simulink model "model_all"  (R2020a)
settings: Solver=VariableStepAuto  StartTime=0.0  StopTime=10.0  RelTol=1e-3
values from neighbouring files (symbols this model uses):
  delta_max = 20    [initialize_all.m]
  ir = 1.7    [initialize_all.m]
  parking_speed = 0.1    [initialize_all.m]
  pr = 1.3    [initialize_all.m]
  TOF_distance_limit = 20    [initialize_all.m]
undefined symbols (not defined in the file or in its folder): denom_drehzahl, num_drehzahl
libraries: robotlib x20, simulink x4, drivingvehiclecontroller x2

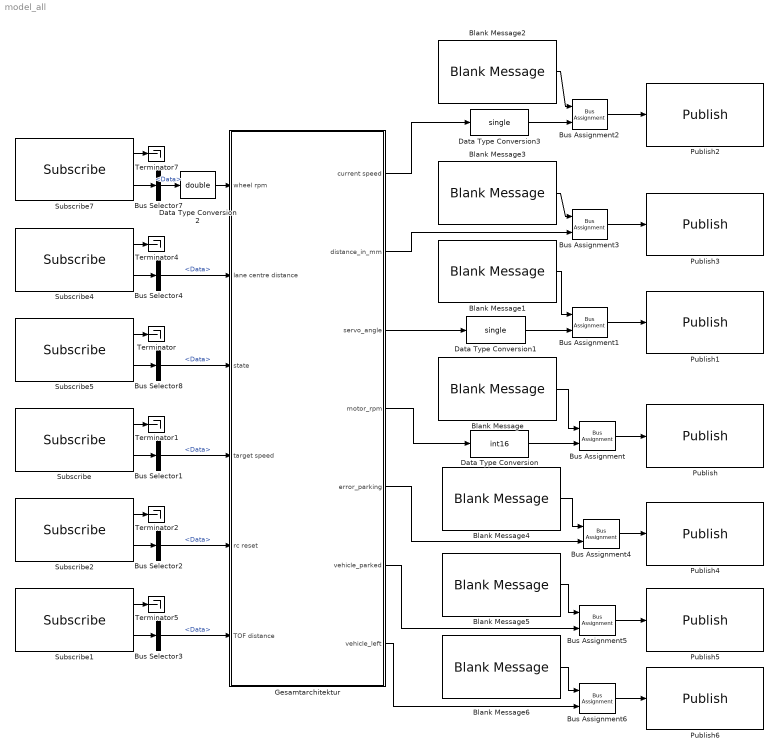
== system model_all ==
  Blank Message : robotlib/Blank Message  messageClass=Message  entityType=std_msgs/Int16  messageType=std_msgs/Int16  SampleTime=inf
  Blank Message1 : robotlib/Blank Message  messageClass=Message  entityType=std_msgs/Float32  messageType=std_msgs/Float32  SampleTime=inf
  Blank Message2 : robotlib/Blank Message  messageClass=Message  entityType=std_msgs/Float32  messageType=std_msgs/Float32  SampleTime=inf
  Blank Message3 : robotlib/Blank Message  messageClass=Message  entityType=std_msgs/Float32  messageType=std_msgs/Float32  SampleTime=inf
  Blank Message4 : robotlib/Blank Message  messageClass=Message  entityType=std_msgs/Bool  messageType=std_msgs/Bool  SampleTime=inf
  Blank Message5 : robotlib/Blank Message  messageClass=Message  entityType=std_msgs/Bool  messageType=std_msgs/Bool  SampleTime=inf
  Blank Message6 : robotlib/Blank Message  messageClass=Message  entityType=std_msgs/Bool  messageType=std_msgs/Bool  SampleTime=inf
  Bus Assignment{,1..6} (7 alike) : BusAssignment  AssignedSignals=Data
  Bus Selector{1..4,7..8} (6 alike) : BusSelector  OutputSignals=Data
  Data Type Conversion : DataTypeConversion  OutDataTypeStr=int16
  Data Type Conversion1 : DataTypeConversion  OutDataTypeStr=single
  Data Type Conversion2 : DataTypeConversion  OutDataTypeStr=double
  Data Type Conversion3 : DataTypeConversion  OutDataTypeStr=single
  Gesamtarchitektur : Subsystem
  Publish : robotlib/Publish  topicSource=Specify your own  topic=/ctl_motorRpm  messageType=std_msgs/Int16  messageQueueLength=1
  Publish1 : robotlib/Publish  topicSource=Specify your own  topic=/ctl_servoAngle  messageType=std_msgs/Float32  messageQueueLength=1
  Publish2 : robotlib/Publish  topicSource=Specify your own  topic=/ctl_velocity  messageType=std_msgs/Float32  messageQueueLength=1
  Publish3 : robotlib/Publish  topicSource=Specify your own  topic=/ctl_distance  messageType=std_msgs/Float32  messageQueueLength=1
  Publish4 : robotlib/Publish  topicSource=Specify your own  topic=/ctl_errorParking  messageType=std_msgs/Bool  messageQueueLength=1
  Publish5 : robotlib/Publish  topicSource=Specify your own  topic=/ctl_parked  messageType=std_msgs/Bool  messageQueueLength=1
  Publish6 : robotlib/Publish  topicSource=Specify your own  topic=/ctl_leavedParkingLot  messageType=std_msgs/Bool  messageQueueLength=1
  Subscribe : robotlib/Subscribe  topicSource=Specify your own  topic=/trj_targetSpeed  messageType=std_msgs/Float32  sampleTime=-1  messageQueueLength=1
  Subscribe1 : robotlib/Subscribe  topicSource=Specify your own  topic=/sns_tof_front  messageType=std_msgs/Float32  sampleTime=-1  messageQueueLength=1
  Subscribe2 : robotlib/Subscribe  topicSource=Specify your own  topic=/akt_rc  messageType=std_msgs/Bool  sampleTime=-1  messageQueueLength=1
  Subscribe4 : robotlib/Subscribe  topicSource=Specify your own  topic=/trj_deltaY  messageType=std_msgs/Float32  sampleTime=-1  messageQueueLength=1
  Subscribe5 : robotlib/Subscribe  topicSource=Specify your own  topic=/state  messageType=std_msgs/Int16  sampleTime=-1  messageQueueLength=1
  Subscribe7 : robotlib/Subscribe  topicSource=Specify your own  topic=/sns_wheelRpm  messageType=std_msgs/Float32  sampleTime=-1  messageQueueLength=1
  Terminator{,1..2,4..5,7} (6 alike) : Terminator
  wires:
  Data Type Conversion/1 -> Bus Assignment/2
  Blank Message/1 -> Bus Assignment/1
  Subscribe/1 -> Terminator1/1
  Bus Assignment/1 -> Publish/1
  Subscribe/2 -> Bus Selector1/1
  Subscribe2/2 -> Bus Selector2/1
  Subscribe2/1 -> Terminator2/1
  Bus Assignment1/1 -> Publish1/1
  Blank Message1/1 -> Bus Assignment1/1
  Data Type Conversion1/1 -> Bus Assignment1/2
  Subscribe4/1 -> Terminator4/1
  Subscribe4/2 -> Bus Selector4/1
  Bus Assignment3/1 -> Publish3/1
  Data Type Conversion3/1 -> Bus Assignment2/2
  Bus Assignment2/1 -> Publish2/1
  Subscribe7/1 -> Terminator7/1
  Blank Message3/1 -> Bus Assignment3/1
  Subscribe7/2 -> Bus Selector7/1
  Blank Message2/1 -> Bus Assignment2/1
  Bus Selector7/1 -> Data Type Conversion2/1  "<Data>"
  Subscribe1/2 -> Bus Selector3/1
  Subscribe1/1 -> Terminator5/1
  Subscribe5/1 -> Terminator/1
  Subscribe5/2 -> Bus Selector8/1
  Bus Assignment4/1 -> Publish4/1
  Blank Message4/1 -> Bus Assignment4/1
  Gesamtarchitektur/5(error_parking) -> Bus Assignment4/2
  Blank Message5/1 -> Bus Assignment5/1
  Bus Assignment5/1 -> Publish5/1
  Gesamtarchitektur/6(vehicle_parked) -> Bus Assignment5/2
  Blank Message6/1 -> Bus Assignment6/1
  Bus Assignment6/1 -> Publish6/1
  Gesamtarchitektur/7(vehicle_left) -> Bus Assignment6/2
  Data Type Conversion2/1 -> Gesamtarchitektur/1(wheel rpm)
  Bus Selector4/1 -> Gesamtarchitektur/2(lane centre distance)  "<Data>"
  Bus Selector8/1 -> Gesamtarchitektur/3(state)  "<Data>"
  Bus Selector1/1 -> Gesamtarchitektur/4(target speed)  "<Data>"
  Bus Selector2/1 -> Gesamtarchitektur/5(rc reset)  "<Data>"
  Bus Selector3/1 -> Gesamtarchitektur/6(TOF distance)  "<Data>"
  Gesamtarchitektur/1(current speed) -> Data Type Conversion3/1
  Gesamtarchitektur/2(distance_in_mm) -> Bus Assignment3/2
  Gesamtarchitektur/3(servo_angle) -> Data Type Conversion1/1
  Gesamtarchitektur/4(motor_rpm) -> Data Type Conversion/1

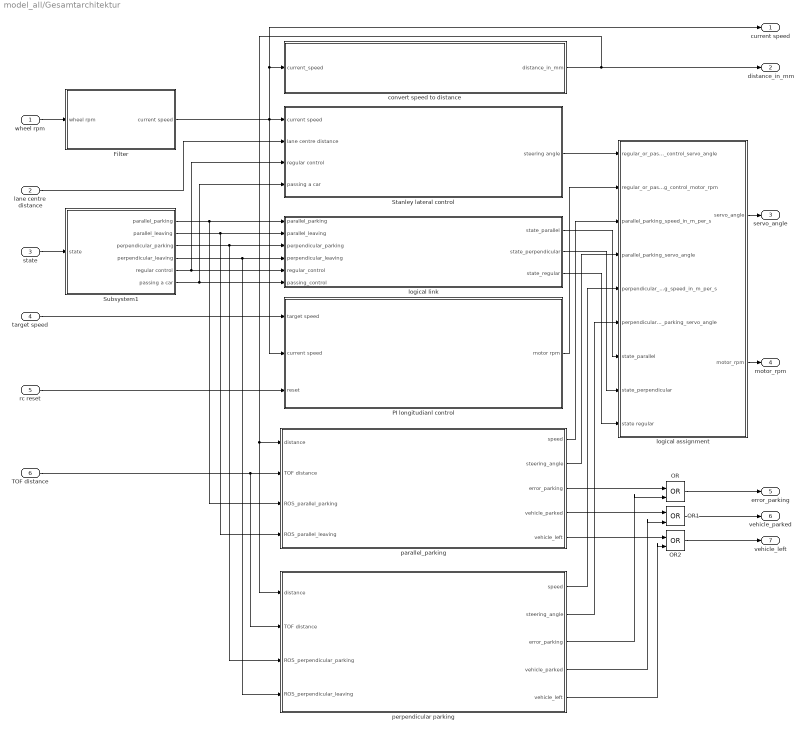
== system model_all/Gesamtarchitektur ==
  wheel rpm : Inport
  lane centre distance : Inport  Port=2
  state : Inport  Port=3
  target speed : Inport  Port=4
  rc reset : Inport  Port=5
  TOF distance : Inport  Port=6
  "Filter " : Subsystem
  OR : Logic  Operator=OR  IconShape=distinctive  AllPortsSameDT=off  OutDataTypeStr=boolean
  OR1 : Logic  Operator=OR  IconShape=distinctive  AllPortsSameDT=off  OutDataTypeStr=boolean
  OR2 : Logic  Operator=OR  IconShape=distinctive  AllPortsSameDT=off  OutDataTypeStr=boolean
  "PI longitudianl control " : Subsystem
  Stanley lateral control : Subsystem
  Subsystem1 : Subsystem
  convert speed to distance : Subsystem
  logical assignment : Subsystem
  logical link : Subsystem
  parallel_parking : Subsystem
  perpendicular parking : Subsystem
  current speed : Outport
  distance_in_mm : Outport  Port=2
  servo_angle : Outport  Port=3
  motor_rpm : Outport  Port=4
  error_parking : Outport  Port=5
  vehicle_parked : Outport  Port=6
  vehicle_left : Outport  Port=7
  wires:
  parallel_parking/1(speed) -> logical assignment/3(parallel_parking_speed_in_m_per_s)
  convert speed to distance/1(distance_in_mm) -> distance_in_mm/1, perpendicular parking/1(distance), parallel_parking/1(distance)
  logical assignment/2(motor_rpm) -> motor_rpm/1
  wheel rpm/1 -> "Filter "/1(wheel rpm)
  TOF distance/1 -> perpendicular parking/2(TOF distance), parallel_parking/2(TOF distance)
  perpendicular parking/1(speed) -> logical assignment/5(perpendicular_parking_speed_in_m_per_s)
  rc reset/1 -> "PI longitudianl control "/3("reset ")
  "Filter "/1(current speed) -> current speed/1, convert speed to distance/1(current_speed), "PI longitudianl control "/2("current speed "), Stanley lateral control/1(current speed)
  Subsystem1/6(passing a car) -> logical link/6(passing_control), Stanley lateral control/4(passing a car)
  state/1 -> Subsystem1/1(state)
  Subsystem1/3(perpendicular_parking) -> perpendicular parking/3(ROS_perpendicular_parking), logical link/3(perpendicular_parking)
  Subsystem1/2(parallel_leaving) -> parallel_parking/4(ROS_parallel_leaving), logical link/2(parallel_leaving)
  Subsystem1/4(perpendicular_leaving) -> logical link/4(perpendicular_leaving), perpendicular parking/4(ROS_perpendicular_leaving)
  Subsystem1/1(parallel_parking) -> parallel_parking/3(ROS_parallel_parking), logical link/1(parallel_parking)
  logical link/2(state_perpendicular) -> logical assignment/8(state_perpendicular)
  Subsystem1/5(regular control) -> Stanley lateral control/3(regular control), logical link/5(regular_control)
  logical link/3(state_regular) -> logical assignment/9(state regular)
  logical link/1(state_parallel) -> logical assignment/7(state_parallel)
  "PI longitudianl control "/1("motor rpm ") -> logical assignment/2(regular_or_passing_control_motor_rpm)
  Stanley lateral control/1(steering angle) -> logical assignment/1(regular_or_passing_control_servo_angle)
  perpendicular parking/2(steering_angle) -> logical assignment/6(perpendicular_parking_servo_angle)
  parallel_parking/2(steering_angle) -> logical assignment/4(parallel_parking_servo_angle)
  logical assignment/1(servo_angle) -> servo_angle/1
  target speed/1 -> "PI longitudianl control "/1("target speed ")
  lane centre distance/1 -> Stanley lateral control/2(lane centre distance)
  perpendicular parking/3(error_parking) -> OR/2
  OR/1 -> error_parking/1
  parallel_parking/3(error_parking) -> OR/1
  OR2/1 -> vehicle_left/1
  perpendicular parking/5(vehicle_left) -> OR2/2
  parallel_parking/5(vehicle_left) -> OR2/1
  perpendicular parking/4(vehicle_parked) -> OR1/2
  OR1/1 -> vehicle_parked/1
  parallel_parking/4(vehicle_parked) -> OR1/1

== system model_all/Gesamtarchitektur/Filter  ==
  wheel rpm : Inport
  Discrete Transfer Fcn : DiscreteTransferFcn  Numerator=num_drehzahl  Denominator=denom_drehzahl
  rpm to 1/s : Gain  Gain=1/60
  wheel radius : Gain  Gain=0.175896
  current speed : Outport
  wires:
  Discrete Transfer Fcn/1 -> wheel radius/1
  wheel rpm/1 -> rpm to 1/s/1
  wheel radius/1 -> current speed/1
  rpm to 1/s/1 -> Discrete Transfer Fcn/1

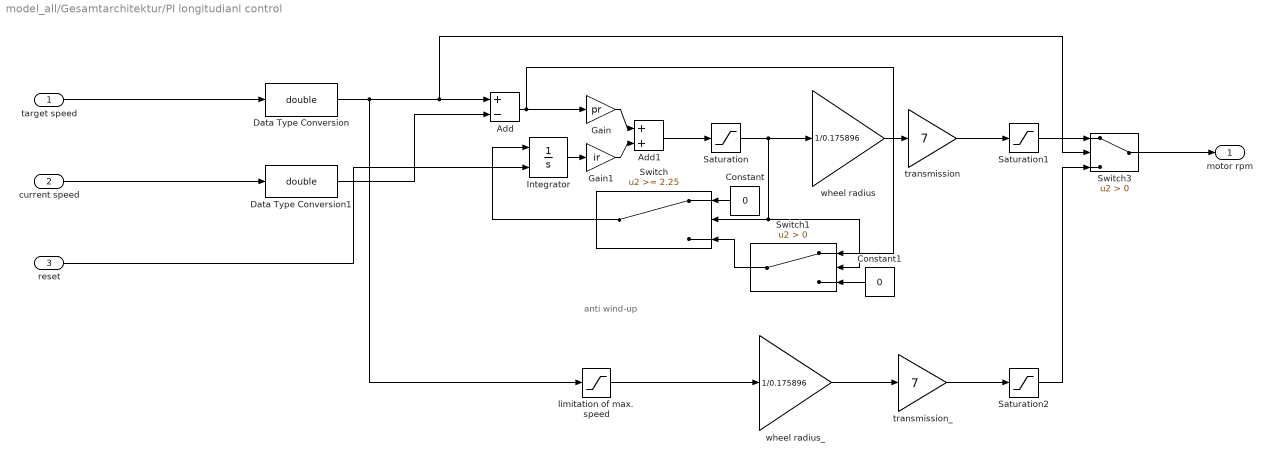
== system model_all/Gesamtarchitektur/PI longitudianl control  ==
  note: anti wind-up
  "target speed " : Inport
  "current speed " : Inport  Port=2
  "reset " : Inport  Port=3
  Add : Sum  Inputs=+-
  Add1 : Sum
  Constant : Constant  Value=0
  Constant1 : Constant  Value=0
  Data Type Conversion : DataTypeConversion  OutDataTypeStr=double
  Data Type Conversion1 : DataTypeConversion  OutDataTypeStr=double
  Gain : Gain  Gain=pr
  Gain1 : Gain  Gain=ir
  Integrator : Integrator  ExternalReset=either
  Saturation : Saturate  UpperLimit=2.3  LowerLimit=0
  Saturation1 : Saturate  UpperLimit=inf  LowerLimit=0
  Saturation2 : Saturate  UpperLimit=0  LowerLimit=-inf
  Switch : Switch  Threshold=2.25
  Switch1 : Switch  Criteria=u2 > Threshold
  Switch3 : Switch  Criteria=u2 > Threshold
  limitation of max. speed : Saturate  UpperLimit=0  LowerLimit=-2.3
  transmission : Gain  Gain=7
  transmission_ : Gain  Gain=7
  wheel radius : Gain  Gain=1/0.175896
  wheel radius_ : Gain  Gain=1/0.175896
  "motor rpm " : Outport
  wires:
  "target speed "/1 -> Data Type Conversion/1
  Data Type Conversion/1 -> limitation of max. speed/1, Switch3/2, Add/1
  "current speed "/1 -> Data Type Conversion1/1
  wheel radius/1 -> transmission/1
  Saturation/1 -> Switch1/2, Switch/2, wheel radius/1
  Add/1 -> Switch1/1, Gain/1
  Integrator/1 -> Gain1/1
  Gain/1 -> Add1/1
  Gain1/1 -> Add1/2
  Add1/1 -> Saturation/1
  Switch/1 -> Integrator/1
  Constant/1 -> Switch/1
  Switch1/1 -> Switch/3
  Constant1/1 -> Switch1/3
  Data Type Conversion1/1 -> Add/2
  Saturation1/1 -> Switch3/1
  transmission/1 -> Saturation1/1
  Saturation2/1 -> Switch3/3
  wheel radius_/1 -> transmission_/1
  transmission_/1 -> Saturation2/1
  limitation of max. speed/1 -> wheel radius_/1
  "reset "/1 -> Integrator/2
  Switch3/1 -> "motor rpm "/1

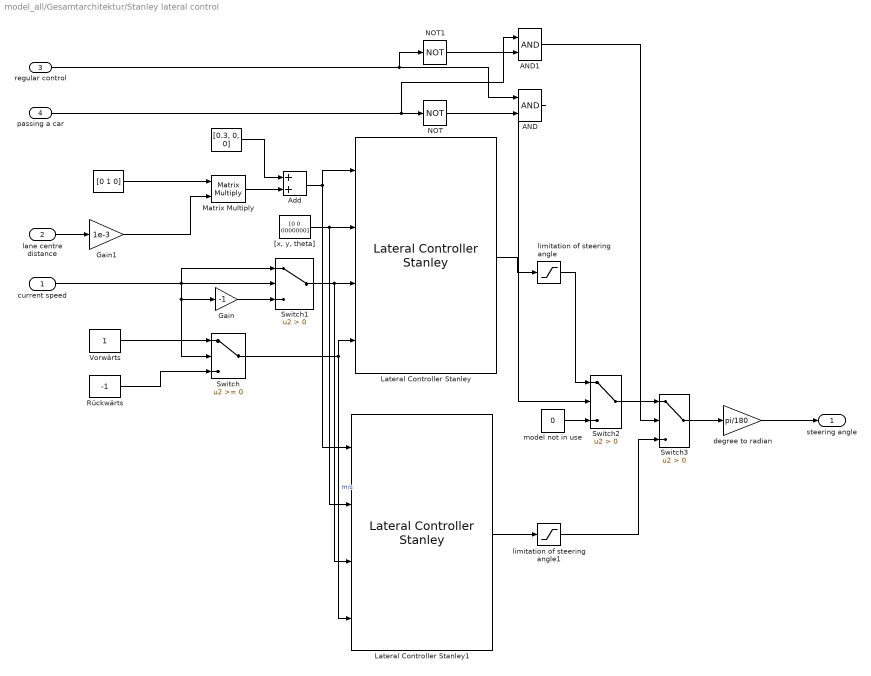
== system model_all/Gesamtarchitektur/Stanley lateral control ==
  current speed : Inport
  lane centre distance : Inport  Port=2
  regular control : Inport  Port=3
  passing a car : Inport  Port=4
  " " : Constant  Value=[0.3, 0, 0]
  " " : Constant  Value=[0 1 0]
  AND : Logic  IconShape=distinctive  AllPortsSameDT=off  OutDataTypeStr=boolean
  AND1 : Logic  IconShape=distinctive  AllPortsSameDT=off  OutDataTypeStr=boolean
  Add : Sum
  Gain : Gain  Gain=-1
  Gain1 : Gain  Gain=1e-3
  Lateral Controller Stanley : drivingvehiclecontroller/Lateral Controller Stanley  ModelType=Kinematic bicycle model  PositionGainF=6  PositionGainR=2.5  YawRateGain=0.2  DelayGain=0.2  VehicleMass=1575  Lf=1.2  Lr=1.6  TireStiffness=19000  Wheelbase=0.25  MaxSteeringAngle=20
  Lateral Controller Stanley1 : drivingvehiclecontroller/Lateral Controller Stanley  ModelType=Kinematic bicycle model  PositionGainF=1  PositionGainR=1  YawRateGain=0.2  DelayGain=0.2  VehicleMass=1575  Lf=1.2  Lr=1.6  TireStiffness=19000  Wheelbase=0.25  MaxSteeringAngle=20
  Matrix Multiply : Product  Multiplication=Matrix(*)
  NOT : Logic  Operator=NOT  IconShape=distinctive  AllPortsSameDT=off  OutDataTypeStr=boolean
  NOT1 : Logic  Operator=NOT  IconShape=distinctive  AllPortsSameDT=off  OutDataTypeStr=boolean
  Rückwärts : Constant  Value=-1
  Switch : Switch
  Switch1 : Switch  Criteria=u2 > Threshold
  Switch2 : Switch  Criteria=u2 > Threshold
  Switch3 : Switch  Criteria=u2 > Threshold
  Vorwärts : Constant
  "[x, y, theta]" : Constant  Value=[0 0 0000000]
  degree to radian : Gain  Gain=pi/180
  limitation of steering angle : Saturate  UpperLimit=20  LowerLimit=-20
  limitation of steering angle1 : Saturate  UpperLimit=20  LowerLimit=-20
  model not in use : Constant  Value=0
  steering angle : Outport
  wires:
  " "/1 -> Add/1
  Add/1 -> Lateral Controller Stanley/1, Lateral Controller Stanley1/1
  Switch1/1 -> Lateral Controller Stanley1/3, Lateral Controller Stanley/3
  current speed/1 -> Switch1/2, Switch1/1, Switch/2, Gain/1
  limitation of steering angle/1 -> Switch2/1
  degree to radian/1 -> steering angle/1
  Matrix Multiply/1 -> Add/2
  "[x, y, theta]"/1 -> Lateral Controller Stanley1/2, Lateral Controller Stanley/2
  lane centre distance/1 -> Gain1/1
  Rückwärts/1 -> Switch/3
  Vorwärts/1 -> Switch/1
  " "/1 -> Matrix Multiply/1
  Switch/1 -> Lateral Controller Stanley/4, Lateral Controller Stanley1/4  "m/s"
  Gain/1 -> Switch1/3
  Lateral Controller Stanley/1 -> limitation of steering angle/1
  Gain1/1 -> Matrix Multiply/2
  Lateral Controller Stanley1/1 -> limitation of steering angle1/1
  NOT/1 -> AND/2
  AND/1 -> Switch2/2
  Switch2/1 -> Switch3/1
  regular control/1 -> NOT1/1, AND/1
  NOT1/1 -> AND1/2
  passing a car/1 -> AND1/1, NOT/1
  AND1/1 -> Switch3/2
  model not in use/1 -> Switch2/3
  limitation of steering angle1/1 -> Switch3/3
  Switch3/1 -> degree to radian/1

== system model_all/Gesamtarchitektur/Subsystem1 ==
  state : Inport
  Switch Case : SwitchCase  CaseConditions={1,2,3,4,5,6}  ShowDefaultCase=off
  parallel_parking : Outport
  parallel_leaving : Outport  Port=2
  perpendicular_parking : Outport  Port=3
  perpendicular_leaving : Outport  Port=4
  regular control : Outport  Port=5
  passing a car : Outport  Port=6
  wires:
  Switch Case/6 -> perpendicular_leaving/1  "perpendicular_leaving"
  state/1 -> Switch Case/1
  Switch Case/5 -> perpendicular_parking/1  "perpendicular_parking"
  Switch Case/4 -> parallel_leaving/1  "parallel_leaving"
  Switch Case/3 -> parallel_parking/1  "parallel_parking"
  Switch Case/2 -> passing a car/1  "passing a car"
  Switch Case/1 -> regular control/1  "regular control"

== system model_all/Gesamtarchitektur/convert speed to distance ==
  current_speed : Inport
  Data Type Conversion4 : DataTypeConversion  OutDataTypeStr=single
  Integrator : Integrator
  distance in mm : Gain  Gain=1000
  distance_in_mm : Outport
  wires:
  current_speed/1 -> Integrator/1
  Data Type Conversion4/1 -> distance in mm/1
  Integrator/1 -> Data Type Conversion4/1
  distance in mm/1 -> distance_in_mm/1

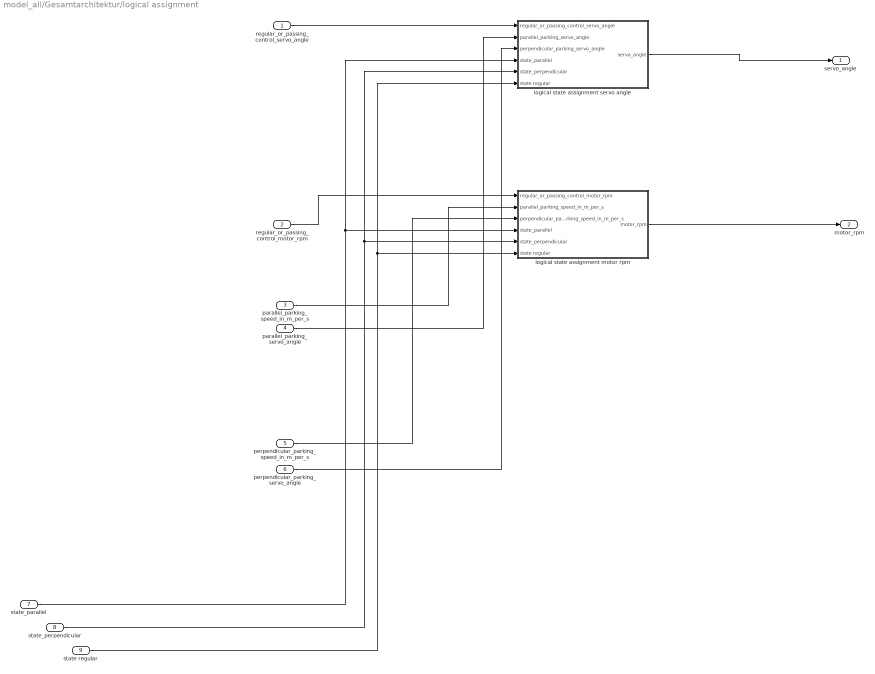
== system model_all/Gesamtarchitektur/logical assignment ==
  regular_or_passing_control_servo_angle : Inport
  regular_or_passing_control_motor_rpm : Inport  Port=2
  parallel_parking_speed_in_m_per_s : Inport  Port=3
  parallel_parking_servo_angle : Inport  Port=4
  perpendicular_parking_speed_in_m_per_s : Inport  Port=5
  perpendicular_parking_servo_angle : Inport  Port=6
  state_parallel : Inport  Port=7
  state_perpendicular : Inport  Port=8
  state regular : Inport  Port=9
  logical state assignment motor rpm : Subsystem
  logical state assignment servo angle : Subsystem
  servo_angle : Outport
  motor_rpm : Outport  Port=2
  wires:
  state regular/1 -> logical state assignment servo angle/6(state regular), logical state assignment motor rpm/6(state regular)
  perpendicular_parking_speed_in_m_per_s/1 -> logical state assignment motor rpm/3(perpendicular_parking_speed_in_m_per_s)
  state_parallel/1 -> logical state assignment motor rpm/4(state_parallel), logical state assignment servo angle/4(state_parallel)
  state_perpendicular/1 -> logical state assignment motor rpm/5(state_perpendicular), logical state assignment servo angle/5(state_perpendicular)
  perpendicular_parking_servo_angle/1 -> logical state assignment servo angle/3(perpendicular_parking_servo_angle)
  logical state assignment motor rpm/1(motor_rpm) -> motor_rpm/1
  regular_or_passing_control_motor_rpm/1 -> logical state assignment motor rpm/1(regular_or_passing_control_motor_rpm)
  parallel_parking_speed_in_m_per_s/1 -> logical state assignment motor rpm/2(parallel_parking_speed_in_m_per_s)
  regular_or_passing_control_servo_angle/1 -> logical state assignment servo angle/1(regular_or_passing_control_servo_angle)
  parallel_parking_servo_angle/1 -> logical state assignment servo angle/2(parallel_parking_servo_angle)
  logical state assignment servo angle/1(servo_angle) -> servo_angle/1

== system model_all/Gesamtarchitektur/logical link ==
  parallel_parking : Inport
  parallel_leaving : Inport  Port=2
  perpendicular_parking : Inport  Port=3
  perpendicular_leaving : Inport  Port=4
  regular_control : Inport  Port=5
  passing_control : Inport  Port=6
  OR3 : Logic  Operator=OR  IconShape=distinctive  AllPortsSameDT=off  OutDataTypeStr=boolean
  OR4 : Logic  Operator=OR  IconShape=distinctive  AllPortsSameDT=off  OutDataTypeStr=boolean
  OR5 : Logic  Operator=OR  IconShape=distinctive  AllPortsSameDT=off  OutDataTypeStr=boolean
  state_parallel : Outport
  state_perpendicular : Outport  Port=2
  state_regular : Outport  Port=3
  wires:
  OR4/1 -> state_perpendicular/1
  perpendicular_leaving/1 -> OR4/2
  OR5/1 -> state_regular/1
  perpendicular_parking/1 -> OR4/1
  parallel_leaving/1 -> OR3/2
  passing_control/1 -> OR5/2
  OR3/1 -> state_parallel/1
  parallel_parking/1 -> OR3/1
  regular_control/1 -> OR5/1

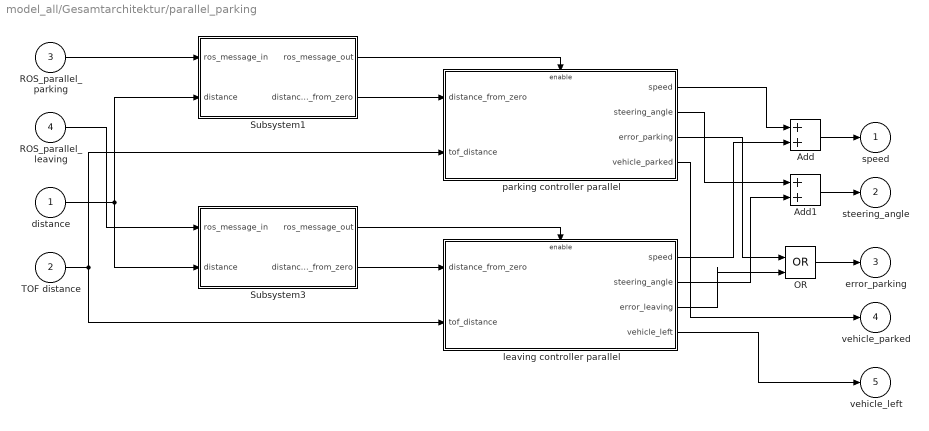
== system model_all/Gesamtarchitektur/parallel_parking ==
  distance : Inport
  TOF distance : Inport  Port=2
  ROS_parallel_parking : Inport  Port=3
  ROS_parallel_leaving : Inport  Port=4
  Add : Sum
  Add1 : Sum
  OR : Logic  Operator=OR  IconShape=distinctive  AllPortsSameDT=off  OutDataTypeStr=boolean
  Subsystem1 : Subsystem
  Subsystem3 : Subsystem
  leaving controller parallel : Subsystem
  parking controller parallel : Subsystem
  speed : Outport
  steering_angle : Outport  Port=2
  error_parking : Outport  Port=3
  vehicle_parked : Outport  Port=4
  vehicle_left : Outport  Port=5
  wires:
  leaving controller parallel/3(error_leaving) -> OR/2
  Add1/1 -> steering_angle/1
  TOF distance/1 -> leaving controller parallel/2(tof_distance), parking controller parallel/2(tof_distance)
  parking controller parallel/3(error_parking) -> OR/1
  distance/1 -> Subsystem3/2(distance), Subsystem1/2(distance)
  parking controller parallel/4("vehicle_parked ") -> vehicle_parked/1
  ROS_parallel_leaving/1 -> Subsystem3/1(ros_message_in)
  parking controller parallel/1(speed) -> Add/1
  leaving controller parallel/4(vehicle_left) -> vehicle_left/1
  Subsystem3/1("ros_message_out ") -> leaving controller parallel/Enable
  Subsystem1/2(distance_from_zero) -> parking controller parallel/1(distance_from_zero)
  Subsystem3/2(distance_from_zero) -> leaving controller parallel/1(distance_from_zero)
  Subsystem1/1("ros_message_out ") -> parking controller parallel/Enable
  ROS_parallel_parking/1 -> Subsystem1/1(ros_message_in)
  leaving controller parallel/2(steering_angle) -> Add1/2
  OR/1 -> error_parking/1
  Add/1 -> speed/1
  leaving controller parallel/1(speed) -> Add/2
  parking controller parallel/2(steering_angle) -> Add1/1

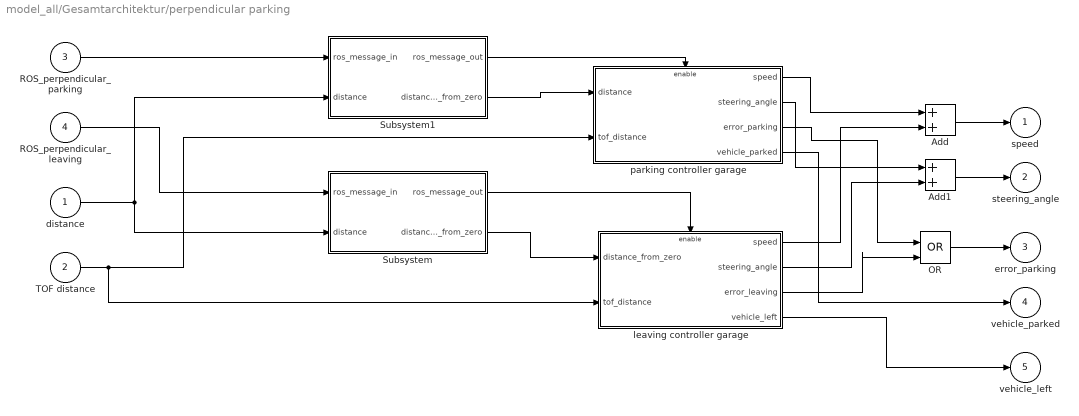
== system model_all/Gesamtarchitektur/perpendicular parking ==
  distance : Inport
  TOF distance : Inport  Port=2
  ROS_perpendicular_parking : Inport  Port=3
  ROS_perpendicular_leaving : Inport  Port=4
  Add : Sum
  Add1 : Sum
  OR : Logic  Operator=OR  IconShape=distinctive  AllPortsSameDT=off  OutDataTypeStr=boolean
  Subsystem : Subsystem
  Subsystem1 : Subsystem
  leaving controller garage : Subsystem
  parking controller garage : Subsystem
  speed : Outport
  steering_angle : Outport  Port=2
  error_parking : Outport  Port=3
  vehicle_parked : Outport  Port=4
  vehicle_left : Outport  Port=5
  wires:
  Subsystem/2(distance_from_zero) -> leaving controller garage/1(distance_from_zero)
  Subsystem1/2(distance_from_zero) -> parking controller garage/1(distance)
  Subsystem1/1("ros_message_out ") -> parking controller garage/Enable
  TOF distance/1 -> parking controller garage/2(tof_distance), leaving controller garage/2(tof_distance)
  parking controller garage/2(steering_angle) -> Add1/1
  Subsystem/1("ros_message_out ") -> leaving controller garage/Enable
  distance/1 -> Subsystem/2(distance), Subsystem1/2(distance)
  leaving controller garage/2(steering_angle) -> Add1/2
  leaving controller garage/3(error_leaving) -> OR/2
  OR/1 -> error_parking/1
  leaving controller garage/4(vehicle_left) -> vehicle_left/1
  leaving controller garage/1(speed) -> Add/2
  Add1/1 -> steering_angle/1
  Add/1 -> speed/1
  parking controller garage/3(error_parking) -> OR/1
  ROS_perpendicular_parking/1 -> Subsystem1/1(ros_message_in)
  parking controller garage/4("vehicle_parked ") -> vehicle_parked/1
  ROS_perpendicular_leaving/1 -> Subsystem/1(ros_message_in)
  parking controller garage/1(speed) -> Add/1

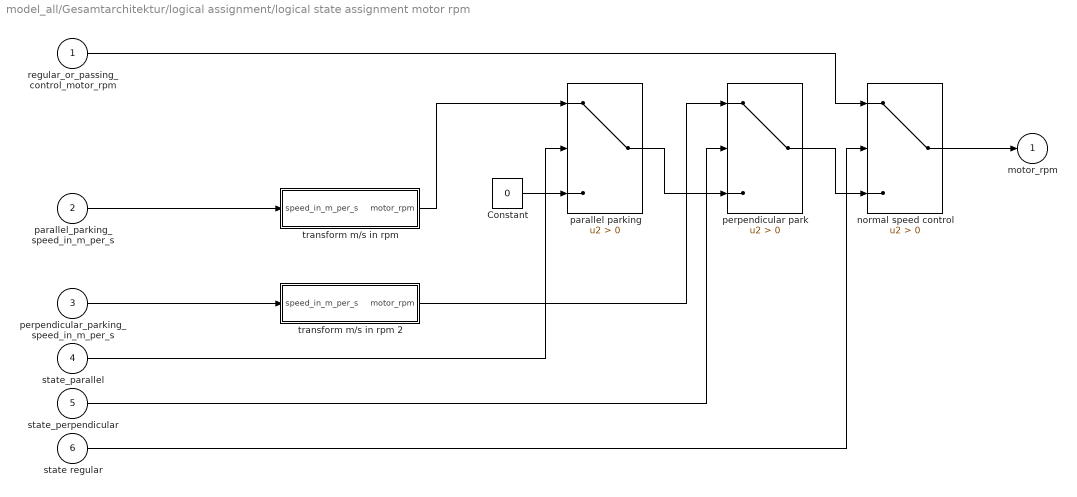
== system model_all/Gesamtarchitektur/logical assignment/logical state assignment motor rpm ==
  regular_or_passing_control_motor_rpm : Inport
  parallel_parking_speed_in_m_per_s : Inport  Port=2
  perpendicular_parking_speed_in_m_per_s : Inport  Port=3
  state_parallel : Inport  Port=4
  state_perpendicular : Inport  Port=5
  state regular : Inport  Port=6
  Constant : Constant  Value=0
  normal speed control : Switch  Criteria=u2 > Threshold
  parallel parking : Switch  Criteria=u2 > Threshold
  perpendicular park : Switch  Criteria=u2 > Threshold
  transform m/s in rpm : Subsystem
  transform m/s in rpm 2 : Subsystem
  motor_rpm : Outport
  wires:
  Constant/1 -> parallel parking/3
  transform m/s in rpm 2/1(motor_rpm) -> perpendicular park/1
  transform m/s in rpm/1(motor_rpm) -> parallel parking/1
  state_perpendicular/1 -> perpendicular park/2
  perpendicular_parking_speed_in_m_per_s/1 -> transform m/s in rpm 2/1(speed_in_m_per_s)
  perpendicular park/1 -> normal speed control/3
  normal speed control/1 -> motor_rpm/1
  regular_or_passing_control_motor_rpm/1 -> normal speed control/1
  state_parallel/1 -> parallel parking/2
  parallel parking/1 -> perpendicular park/3
  parallel_parking_speed_in_m_per_s/1 -> transform m/s in rpm/1(speed_in_m_per_s)
  state regular/1 -> normal speed control/2

== system model_all/Gesamtarchitektur/logical assignment/logical state assignment servo angle ==
  regular_or_passing_control_servo_angle : Inport
  parallel_parking_servo_angle : Inport  Port=2
  perpendicular_parking_servo_angle : Inport  Port=3
  state_parallel : Inport  Port=4
  state_perpendicular : Inport  Port=5
  state regular : Inport  Port=6
  Constant : Constant  Value=0
  normal servo control : Switch  Criteria=u2 > Threshold
  parallel parking servo : Switch  Criteria=u2 > Threshold
  perpendicular park servo : Switch  Criteria=u2 > Threshold
  servo_angle : Outport
  wires:
  Constant/1 -> parallel parking servo/3
  perpendicular_parking_servo_angle/1 -> perpendicular park servo/1
  parallel_parking_servo_angle/1 -> parallel parking servo/1
  state_perpendicular/1 -> perpendicular park servo/2
  perpendicular park servo/1 -> normal servo control/3
  normal servo control/1 -> servo_angle/1
  regular_or_passing_control_servo_angle/1 -> normal servo control/1
  state_parallel/1 -> parallel parking servo/2
  parallel parking servo/1 -> perpendicular park servo/3
  state regular/1 -> normal servo control/2

== system model_all/Gesamtarchitektur/parallel_parking/Subsystem1 ==
  ros_message_in : Inport
  distance : Inport  Port=2
  Delay : Delay  DelayLength=1
  "Detect Rise Positive " : simulink/Logic and Bit Operations/Detect Rise Positive  vinit=0  OutDataTypeStr=boolean
  Subtract : Sum  Inputs=+-
  Switch : Switch  Criteria=u2 ~= 0
  "ros_message_out " : Outport
  distance_from_zero : Outport  Port=2
  wires:
  ros_message_in/1 -> "Detect Rise Positive "/1, "ros_message_out "/1
  Delay/1 -> Switch/3
  Subtract/1 -> distance_from_zero/1
  distance/1 -> Switch/1, Subtract/1
  Switch/1 -> Subtract/2, Delay/1
  "Detect Rise Positive "/1 -> Switch/2

== system model_all/Gesamtarchitektur/parallel_parking/Subsystem3 ==
  ros_message_in : Inport
  distance : Inport  Port=2
  Delay : Delay  DelayLength=1
  "Detect Rise Positive " : simulink/Logic and Bit Operations/Detect Rise Positive  vinit=0  OutDataTypeStr=boolean
  Subtract : Sum  Inputs=+-
  Switch : Switch  Criteria=u2 ~= 0
  "ros_message_out " : Outport
  distance_from_zero : Outport  Port=2
  wires:
  ros_message_in/1 -> "Detect Rise Positive "/1, "ros_message_out "/1
  Delay/1 -> Switch/3
  Subtract/1 -> distance_from_zero/1
  distance/1 -> Switch/1, Subtract/1
  Switch/1 -> Subtract/2, Delay/1
  "Detect Rise Positive "/1 -> Switch/2

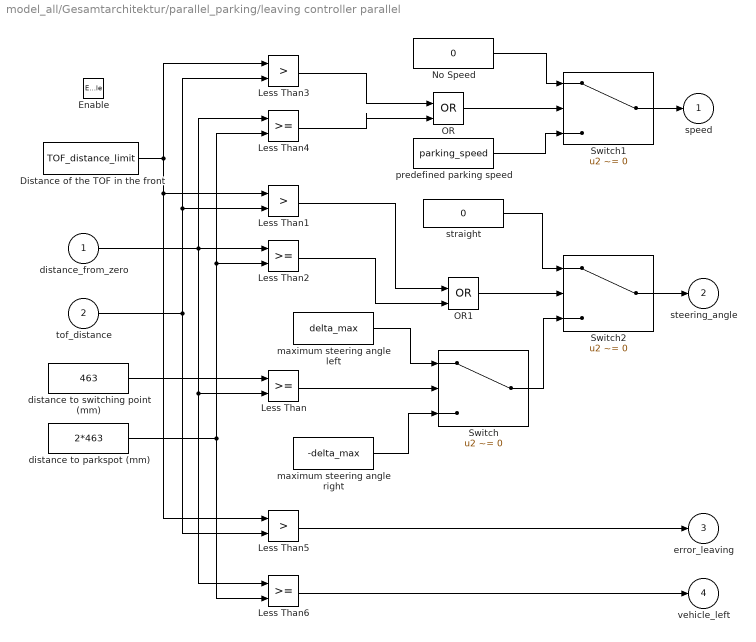
== system model_all/Gesamtarchitektur/parallel_parking/leaving controller parallel ==
  distance_from_zero : Inport
  tof_distance : Inport  Port=2
  Enable : EnablePort
  "Distance of the TOF in the front " : Constant  Value=TOF_distance_limit
  Less Than{,2,4,6} (4 alike) : RelationalOperator  OutDataTypeStr=boolean  RndMeth=Simplest
  Less Than1 : RelationalOperator  Operator=>  OutDataTypeStr=boolean  RndMeth=Simplest
  Less Than3 : RelationalOperator  Operator=>  OutDataTypeStr=boolean  RndMeth=Simplest
  Less Than5 : RelationalOperator  Operator=>  OutDataTypeStr=boolean  RndMeth=Simplest
  No Speed : Constant  Value=0
  OR : Logic  Operator=OR  IconShape=distinctive  AllPortsSameDT=off  OutDataTypeStr=boolean
  OR1 : Logic  Operator=OR  IconShape=distinctive  AllPortsSameDT=off  OutDataTypeStr=boolean
  Switch : Switch  Criteria=u2 ~= 0  Threshold=1079  OutDataTypeStr=single
  Switch1 : Switch  Criteria=u2 ~= 0  Threshold=1377  OutDataTypeStr=single
  Switch2 : Switch  Criteria=u2 ~= 0  Threshold=1079  OutDataTypeStr=single
  distance to parkspot (mm) : Constant  Value=2*463
  "distance to switching point (mm) " : Constant  Value=463
  maximum steering angle left : Constant  Value=delta_max
  maximum steering angle right : Constant  Value=-delta_max
  predefined parking speed : Constant  Value=parking_speed
  straight : Constant  Value=0
  speed : Outport
  steering_angle : Outport  Port=2
  error_leaving : Outport  Port=3
  vehicle_left : Outport  Port=4
  wires:
  maximum steering angle right/1 -> Switch/3
  Less Than/1 -> Switch/2
  predefined parking speed/1 -> Switch1/3
  No Speed/1 -> Switch1/1
  Switch/1 -> Switch2/3
  OR/1 -> Switch1/2
  Switch1/1 -> speed/1
  maximum steering angle left/1 -> Switch/1
  Switch2/1 -> steering_angle/1
  straight/1 -> Switch2/1
  "distance to switching point (mm) "/1 -> Less Than/1
  distance_from_zero/1 -> Less Than6/1, Less Than/2, Less Than2/1, Less Than4/1
  OR1/1 -> Switch2/2
  tof_distance/1 -> Less Than5/2, Less Than1/2, Less Than3/2
  "Distance of the TOF in the front "/1 -> Less Than3/1, Less Than5/1, Less Than1/1
  distance to parkspot (mm)/1 -> Less Than4/2, Less Than2/2, Less Than6/2
  Less Than2/1 -> OR1/2
  Less Than1/1 -> OR1/1
  Less Than3/1 -> OR/1
  Less Than4/1 -> OR/2
  Less Than6/1 -> vehicle_left/1
  Less Than5/1 -> error_leaving/1

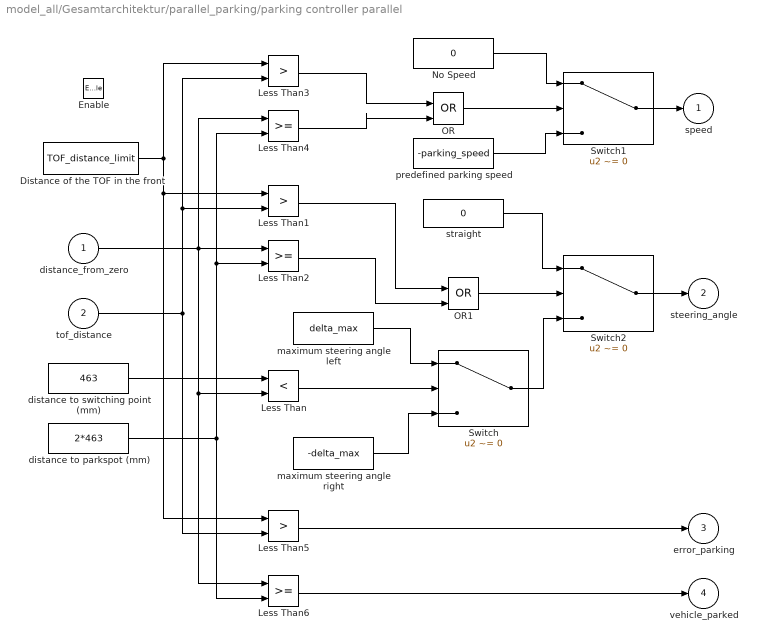
== system model_all/Gesamtarchitektur/parallel_parking/parking controller parallel ==
  distance_from_zero : Inport
  tof_distance : Inport  Port=2
  Enable : EnablePort
  "Distance of the TOF in the front " : Constant  Value=TOF_distance_limit
  Less Than : RelationalOperator  Operator=<  OutDataTypeStr=boolean  RndMeth=Simplest
  Less Than1 : RelationalOperator  Operator=>  OutDataTypeStr=boolean  RndMeth=Simplest
  Less Than2 : RelationalOperator  OutDataTypeStr=boolean  RndMeth=Simplest
  Less Than3 : RelationalOperator  Operator=>  OutDataTypeStr=boolean  RndMeth=Simplest
  Less Than4 : RelationalOperator  OutDataTypeStr=boolean  RndMeth=Simplest
  Less Than5 : RelationalOperator  Operator=>  OutDataTypeStr=boolean  RndMeth=Simplest
  Less Than6 : RelationalOperator  OutDataTypeStr=boolean  RndMeth=Simplest
  No Speed : Constant  Value=0
  OR : Logic  Operator=OR  IconShape=distinctive  AllPortsSameDT=off  OutDataTypeStr=boolean
  OR1 : Logic  Operator=OR  IconShape=distinctive  AllPortsSameDT=off  OutDataTypeStr=boolean
  Switch : Switch  Criteria=u2 ~= 0  Threshold=1079  OutDataTypeStr=single
  Switch1 : Switch  Criteria=u2 ~= 0  Threshold=1377  OutDataTypeStr=single
  Switch2 : Switch  Criteria=u2 ~= 0  Threshold=1079  OutDataTypeStr=single
  distance to parkspot (mm) : Constant  Value=2*463
  "distance to switching point (mm) " : Constant  Value=463
  maximum steering angle left : Constant  Value=delta_max
  maximum steering angle right : Constant  Value=-delta_max
  predefined parking speed : Constant  Value=-parking_speed
  straight : Constant  Value=0
  speed : Outport
  steering_angle : Outport  Port=2
  error_parking : Outport  Port=3
  "vehicle_parked " : Outport  Port=4
  wires:
  maximum steering angle right/1 -> Switch/3
  Less Than/1 -> Switch/2
  predefined parking speed/1 -> Switch1/3
  No Speed/1 -> Switch1/1
  Switch/1 -> Switch2/3
  OR/1 -> Switch1/2
  Switch1/1 -> speed/1
  maximum steering angle left/1 -> Switch/1
  Switch2/1 -> steering_angle/1
  straight/1 -> Switch2/1
  "distance to switching point (mm) "/1 -> Less Than/1
  distance_from_zero/1 -> Less Than6/1, Less Than/2, Less Than2/1, Less Than4/1
  OR1/1 -> Switch2/2
  tof_distance/1 -> Less Than5/2, Less Than1/2, Less Than3/2
  "Distance of the TOF in the front "/1 -> Less Than3/1, Less Than5/1, Less Than1/1
  distance to parkspot (mm)/1 -> Less Than4/2, Less Than2/2, Less Than6/2
  Less Than2/1 -> OR1/2
  Less Than1/1 -> OR1/1
  Less Than3/1 -> OR/1
  Less Than4/1 -> OR/2
  Less Than6/1 -> "vehicle_parked "/1
  Less Than5/1 -> error_parking/1

== system model_all/Gesamtarchitektur/perpendicular parking/Subsystem ==
  ros_message_in : Inport
  distance : Inport  Port=2
  Delay : Delay  DelayLength=1
  "Detect Rise Positive " : simulink/Logic and Bit Operations/Detect Rise Positive  vinit=0  OutDataTypeStr=boolean
  Subtract : Sum  Inputs=+-
  Switch : Switch  Criteria=u2 ~= 0
  "ros_message_out " : Outport
  distance_from_zero : Outport  Port=2
  wires:
  ros_message_in/1 -> "Detect Rise Positive "/1, "ros_message_out "/1
  Delay/1 -> Switch/3
  Subtract/1 -> distance_from_zero/1
  distance/1 -> Switch/1, Subtract/1
  Switch/1 -> Subtract/2, Delay/1
  "Detect Rise Positive "/1 -> Switch/2

== system model_all/Gesamtarchitektur/perpendicular parking/Subsystem1 ==
  ros_message_in : Inport
  distance : Inport  Port=2
  Delay : Delay  DelayLength=1
  "Detect Rise Positive " : simulink/Logic and Bit Operations/Detect Rise Positive  vinit=0  OutDataTypeStr=boolean
  Subtract : Sum  Inputs=+-
  Switch : Switch  Criteria=u2 ~= 0
  "ros_message_out " : Outport
  distance_from_zero : Outport  Port=2
  wires:
  ros_message_in/1 -> "Detect Rise Positive "/1, "ros_message_out "/1
  Delay/1 -> Switch/3
  Subtract/1 -> distance_from_zero/1
  distance/1 -> Switch/1, Subtract/1
  Switch/1 -> Subtract/2, Delay/1
  "Detect Rise Positive "/1 -> Switch/2

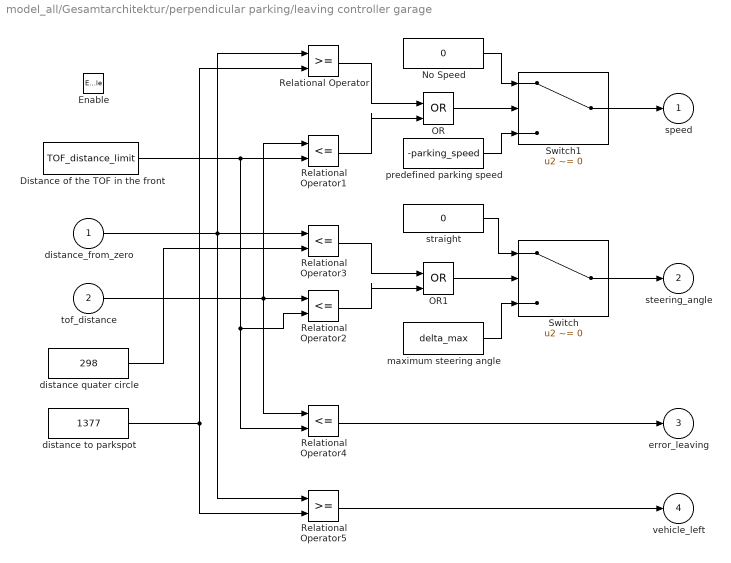
== system model_all/Gesamtarchitektur/perpendicular parking/leaving controller garage ==
  distance_from_zero : Inport
  tof_distance : Inport  Port=2
  Enable : EnablePort
  "Distance of the TOF in the front " : Constant  Value=TOF_distance_limit
  No Speed : Constant  Value=0
  OR : Logic  Operator=OR  IconShape=distinctive  AllPortsSameDT=off  OutDataTypeStr=boolean
  OR1 : Logic  Operator=OR  IconShape=distinctive  AllPortsSameDT=off  OutDataTypeStr=boolean
  Relational Operator : RelationalOperator  OutDataTypeStr=boolean  RndMeth=Simplest
  Relational Operator{1..4} (4 alike) : RelationalOperator  Operator=<=  OutDataTypeStr=boolean  RndMeth=Simplest
  Relational Operator5 : RelationalOperator  OutDataTypeStr=boolean  RndMeth=Simplest
  Switch : Switch  Criteria=u2 ~= 0  Threshold=1079  OutDataTypeStr=single
  Switch1 : Switch  Criteria=u2 ~= 0  Threshold=1377  OutDataTypeStr=single
  "distance quater circle " : Constant  Value=298
  distance to parkspot : Constant  Value=1377
  maximum steering angle : Constant  Value=delta_max
  predefined parking speed : Constant  Value=-parking_speed
  straight : Constant  Value=0
  speed : Outport
  steering_angle : Outport  Port=2
  error_leaving : Outport  Port=3
  vehicle_left : Outport  Port=4
  wires:
  Switch1/1 -> speed/1
  Switch/1 -> steering_angle/1
  straight/1 -> Switch/1
  maximum steering angle/1 -> Switch/3
  No Speed/1 -> Switch1/1
  predefined parking speed/1 -> Switch1/3
  Relational Operator/1 -> OR/1
  OR/1 -> Switch1/2
  Relational Operator1/1 -> OR/2
  tof_distance/1 -> Relational Operator4/1, Relational Operator2/1, Relational Operator1/1
  Relational Operator2/1 -> OR1/2
  "distance quater circle "/1 -> Relational Operator3/2
  Relational Operator3/1 -> OR1/1
  OR1/1 -> Switch/2
  "Distance of the TOF in the front "/1 -> Relational Operator4/2, Relational Operator2/2, Relational Operator1/2
  Relational Operator4/1 -> error_leaving/1
  distance_from_zero/1 -> Relational Operator/1, Relational Operator5/1, Relational Operator3/1
  distance to parkspot/1 -> Relational Operator5/2, Relational Operator/2
  Relational Operator5/1 -> vehicle_left/1

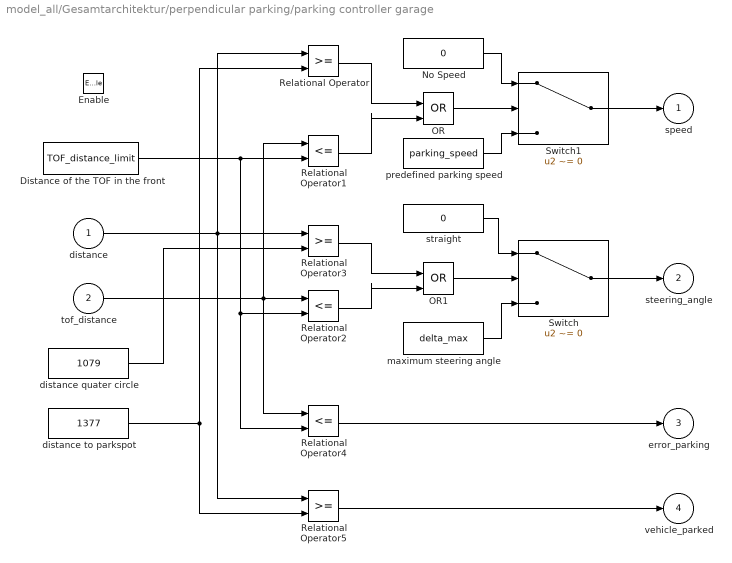
== system model_all/Gesamtarchitektur/perpendicular parking/parking controller garage ==
  distance : Inport
  tof_distance : Inport  Port=2
  Enable : EnablePort
  "Distance of the TOF in the front " : Constant  Value=TOF_distance_limit
  No Speed : Constant  Value=0
  OR : Logic  Operator=OR  IconShape=distinctive  AllPortsSameDT=off  OutDataTypeStr=boolean
  OR1 : Logic  Operator=OR  IconShape=distinctive  AllPortsSameDT=off  OutDataTypeStr=boolean
  Relational Operator : RelationalOperator  OutDataTypeStr=boolean  RndMeth=Simplest
  Relational Operator1 : RelationalOperator  Operator=<=  OutDataTypeStr=boolean  RndMeth=Simplest
  Relational Operator2 : RelationalOperator  Operator=<=  OutDataTypeStr=boolean  RndMeth=Simplest
  Relational Operator3 : RelationalOperator  OutDataTypeStr=boolean  RndMeth=Simplest
  Relational Operator4 : RelationalOperator  Operator=<=  OutDataTypeStr=boolean  RndMeth=Simplest
  Relational Operator5 : RelationalOperator  OutDataTypeStr=boolean  RndMeth=Simplest
  Switch : Switch  Criteria=u2 ~= 0  Threshold=1079  OutDataTypeStr=single
  Switch1 : Switch  Criteria=u2 ~= 0  Threshold=1377  OutDataTypeStr=single
  "distance quater circle " : Constant  Value=1079
  distance to parkspot : Constant  Value=1377
  maximum steering angle : Constant  Value=delta_max
  predefined parking speed : Constant  Value=parking_speed
  straight : Constant  Value=0
  speed : Outport
  steering_angle : Outport  Port=2
  error_parking : Outport  Port=3
  "vehicle_parked " : Outport  Port=4
  wires:
  Switch1/1 -> speed/1
  Switch/1 -> steering_angle/1
  straight/1 -> Switch/1
  maximum steering angle/1 -> Switch/3
  No Speed/1 -> Switch1/1
  predefined parking speed/1 -> Switch1/3
  Relational Operator/1 -> OR/1
  OR/1 -> Switch1/2
  Relational Operator1/1 -> OR/2
  tof_distance/1 -> Relational Operator4/1, Relational Operator2/1, Relational Operator1/1
  Relational Operator2/1 -> OR1/2
  "distance quater circle "/1 -> Relational Operator3/2
  Relational Operator3/1 -> OR1/1
  OR1/1 -> Switch/2
  "Distance of the TOF in the front "/1 -> Relational Operator4/2, Relational Operator2/2, Relational Operator1/2
  Relational Operator4/1 -> error_parking/1
  distance/1 -> Relational Operator/1, Relational Operator5/1, Relational Operator3/1
  distance to parkspot/1 -> Relational Operator5/2, Relational Operator/2
  Relational Operator5/1 -> "vehicle_parked "/1

== system model_all/Gesamtarchitektur/logical assignment/logical state assignment motor rpm/transform m//s in rpm ==
  speed_in_m_per_s : Inport
  Saturation2 : Saturate  UpperLimit=0  LowerLimit=-inf
  transmission_ : Gain  Gain=7
  wheel radius_ : Gain  Gain=1/0.175896
  motor_rpm : Outport
  wires:
  transmission_/1 -> Saturation2/1
  wheel radius_/1 -> transmission_/1
  Saturation2/1 -> motor_rpm/1
  speed_in_m_per_s/1 -> wheel radius_/1

== system model_all/Gesamtarchitektur/logical assignment/logical state assignment motor rpm/transform m//s in rpm 2 ==
  speed_in_m_per_s : Inport
  Saturation2 : Saturate  UpperLimit=0  LowerLimit=-inf
  transmission_ : Gain  Gain=7
  wheel radius_ : Gain  Gain=1/0.175896
  motor_rpm : Outport
  wires:
  transmission_/1 -> Saturation2/1
  wheel radius_/1 -> transmission_/1
  Saturation2/1 -> motor_rpm/1
  speed_in_m_per_s/1 -> wheel radius_/1
